simulink model "EKF_sim"  (R2020a)
settings: Solver=VariableStepAuto  StartTime=0.0  StopTime=257  RelTol=1e-3
values from neighbouring files (symbols this model uses):
  acc_variance = 4.8e-2    (= 0.048)    [init.m]
  bias_acc_variance = 4e-14    [init.m]
  bias_gyro_variance = 4e-14    [init.m]
  Delta2 = [260.168 -23.8158 1.64305]    [init.m]
  DT = EKF_DT    (= 0.01)    [init.m]
  EKF_DT = 0.01    [init.m]
  g = 9.81    [init.m]
  GPS_variance = 5    [init.m]
  gyro_variance = 4.8e-6    (= 4.8e-06)    [init.m]
  h0 = 38.8887000000000000    (= 38.8887)    [init.m]
  head_variance = 5e-2    (= 0.05)    [init.m]
  init_time = 4    [init.m]
  lambda_xa = 1e-4    (= 0.0001)    [init.m]
  lambda_xg = 1e-3    (= 0.001)    [init.m]
  lat0 = 36.7144590750000006    (= 36.714459075)    [init.m]
  lon0 = -4.4789588283333330    (= -4.47895882833)    [init.m]
  SHOE_buffer_N = 100    [init.m]
  SHOE_threshold = 2000    [init.m]
  t1_end = 100    [init.m]
  t1_start = 90    [init.m]
  t2_end = 193    [init.m]
  t2_start = 183    [init.m]
  t3_end = 213    [init.m]
  t3_start = 203    [init.m]
  t4_end = 244    [init.m]
  t4_start = 237    [init.m]
  type_of_GPS = 1    [init.m]
  vel_variance = 1e-2    (= 0.01)    [init.m]
  zero_vel_period = 0.1    [init.m]
(part 2 of 5)

== matlab function EKF_sim/EKF_nb/System Prediction/prediction_step ==
  data: x0 input; x_k output; P0 input; x_k_1 input size=16 1; P_k_1 input size=16 16; yg input; ya input; U input; P_k output size=16 16; DT parameter; g parameter; flag_init input; flag_init_ output
% --------------------         prediction           -------------------- %
%{
% This function computes the prediction step of the Kalman Filter. After 
% the initialization of the system, at each period the state vector is 
% updated, related to the prediction function and the measurement by the 
% inertial sensors (gyroscope and accelerometer). The covariance matrix P 
% is also updated.

% Input:
%     x0         : initial vector state
%     P0         : initial matrix P
%     x_k_1      : state vector before prediction step
%     P_k_1      : matrix P before prediction step
%     yg         : gyroscope measurement
%     ya         : accelerometer measurement
%     U          : covariance Matrix of input sensor
%     DT         : period of EKF system
%     g          : gravity acceleration
%     flag_init  : flag for initialization task

% Output:
%     x_k        : state vector after prediction step
%     P_k        : matrix P after prediction step
%     flag_init_ : flag for initialization task

% State vector x = [q w r v a]' [16x1]:
% q  = [q1 q2 q3 q4]     unit quaternion representing the attitude (1 2 3 4)
% w  = [wx wy wz]        angular velocity (5 6 7)
% r  = [rx ry rz]        position (NED)(8 9 10)
% v  = [vx vy vz]        linear velocity (NED) (11 12 13)
% a  = [ax ay az]        linear acceleration (NED) (14 15 16)
 
% Prediction model functions:
% fq = q * q(w*DT)
% fw = yg;
% fr = r + v*DT + a*DT*DT/2;
% fv = v + a*DT;
% fa = Rnb*ya + [0;0;g];

% P_k = Fx*P_k_1*Fx' + Fu*U*Fu'
 
% U = [gyro_variance(3x3),            0          
%        0                     acc_variance(3x3)]

% See 'calcolo_matrice_F_nb.m' for the exact calculation of matrices Fx and Fu
% These matrices are calculated offline, so note that if same parameters of 
% the system change, these matrices need to be changed.
%}
%%
function [x_k,  P_k, flag_init_] = prediction(x0, P0, x_k_1, P_k_1, ...
                                          yg, ya,...
                                          U, DT, g, flag_init)
    x_k = zeros(16,1);
    P_k = zeros(16,16);
    flag_init_ = flag_init;
    if flag_init ~= 0           %initialization check
        if flag_init == 1
            x_k_1 = x0;
            P_k_1 = P0;
            flag_init_ = 2;     %set flag=2 so the initialization is done
        end                     %one time only
        
        % Prediction Step
        [q_k_1,~,r_k_1,v_k_1,~] = extract_var(x_k_1);
        
        w_k  = yg;                                      %Velocity Rotation update with no bias compensation
        w_DT = (w_k*DT);                                %Angular displacement in DT time interval
        q_w  = new_q(w_DT(1),w_DT(2),w_DT(3));                        
        q    = q_product(q_k_1,q_w);                    %Rotations composition
        norm = (q(1)^2 + q(2)^2 + q(3)^2 + q(4)^2)^0.5;
        q_k  = q/norm;                                  %Normalize new quaternion
        Rnb  = fromq2rot(q_k(1),q_k(2),q_k(3),q_k(4));
       
        a_k  = Rnb*ya + [0;0;g];                        %Acceleration Update with no bias compensation
        v_k  = v_k_1 + a_k*DT;                          %Velocity update
        r_k  = r_k_1 + v_k*DT + a_k*DT*DT/2;            %Position update (origin of body frame)
        
        x_k = compact_var(q_k, w_k, r_k, v_k, a_k);          
        
        Fu = calcolo_Fu(q_k(1),q_k(2),q_k(3),q_k(4));
        Fx = calcolo_Fx(q_k(1),q_k(2),q_k(3),q_k(4),w_k(1),w_k(2),w_k(3),ya(1),ya(2),ya(3));
        P_k = Fx*P_k_1*Fx' + Fu*U*Fu';                  %Matrix P Update           
    end
end

%% Auxiliary Functions
% This function extracts single variables from the state vector
function [q, w, r, v, a] = extract_var(x)
    q  = x(1:4);
    w  = x(5:7);
    r  = x(8:10);
    v  = x(11:13);
    a  = x(14:16);
end

% This function compacts single variables into the state vector
function x = compact_var(q, w, r, v, a)
    x = zeros(16,1);
    x(1:4)   = q;
    x(5:7)   = w;
    x(8:10) =  r;
    x(11:13) = v;
    x(14:16) = a;
end

% This function computes the body-to-nav rotation matrix from quaternion
function rot = fromq2rot(q1,q2,q3,q4)
    rot = [q1^2+q2^2-q3^2-q4^2, 2*(q2*q3-q1*q4), 2*(q1*q3+q2*q4); ...
           2*(q2*q3+q1*q4), q1^2-q2^2+q3^2-q4^2, 2*(q3*q4-q1*q2); ...
           2*(q2*q4-q1*q3), 2*(q1*q2+q3*q4), q1^2-q2^2-q3^2+q4^2];
end

% This function create a quaternion from Euler's angle [Yaw,Pitch,Roll]
function q = new_q(yaw,pitch,roll)
    q = zeros(1,4);
    q(1) = cos(roll/2) * cos(pitch/2) * cos(yaw/2) + sin(roll/2) * sin(pitch/2) * sin(yaw/2);
    q(2) = sin(roll/2) * cos(pitch/2) * cos(yaw/2) - cos(roll/2) * sin(pitch/2) * sin(yaw/2);
    q(3) = cos(roll/2) * sin(pitch/2) * cos(yaw/2) + sin(roll/2) * cos(pitch/2) * sin(yaw/2);
    q(4) = cos(roll/2) * cos(pitch/2) * sin(yaw/2) - sin(roll/2) * sin(pitch/2) * cos(yaw/2);
    
end

% This function computes the product between two quaternion
function q = q_product(a,b)
    q = zeros(1,4);
    q(1) = b(1)*a(1) - b(2)*a(2) - b(3)*a(3) - b(4)*a(4);
    q(2) = b(1)*a(2) + b(2)*a(1) - b(3)*a(4) + b(4)*a(3);
    q(3) = b(1)*a(3) + b(2)*a(4) + b(3)*a(1) - b(4)*a(2);
    q(4) = b(1)*a(4) - b(2)*a(3) + b(3)*a(2) + b(4)*a(1);
end
%%
% These functions calculate the Fx and Fu matrices. 
% See 'calcolo_matrice_F_nb.m' for the symbolic calculation used
function Fx = calcolo_Fx(q1,q2,q3,q4,w_yaw,w_pitch,w_roll,ya1,ya2,ya3)
Fx =[(cos(w_pitch/200)*cos(w_roll/200)*cos(w_yaw/200) + sin(w_pitch/200)*sin(w_roll/200)*sin(w_yaw/200))/(q1^2 + q2^2 + q3^2 + q4^2)^(1/2) + (q1*(q2*(cos(w_pitch/200)*cos(w_yaw/200)*sin(w_roll/200) - cos(w_roll/200)*sin(w_pitch/200)*sin(w_yaw/200)) - q1*(cos(w_pitch/200)*cos(w_roll/200)*cos(w_yaw/200) + sin(w_pitch/200)*sin(w_roll/200)*sin(w_yaw/200)) + q3*(cos(w_roll/200)*cos(w_yaw/200)*sin(w_pitch/200) + cos(w_pitch/200)*sin(w_roll/200)*sin(w_yaw/200)) + q4*(cos(w_pitch/200)*cos(w_roll/200)*sin(w_yaw/200) - cos(w_yaw/200)*sin(w_pitch/200)*sin(w_roll/200))))/(q1^2 + q2^2 + q3^2 + q4^2)^(3/2),   (q2*(q2*(cos(w_pitch/200)*cos(w_yaw/200)*sin(w_roll/200) - cos(w_roll/200)*sin(w_pitch/200)*sin(w_yaw/200)) - q1*(cos(w_pitch/200)*cos(w_roll/200)*cos(w_yaw/200) + sin(w_pitch/200)*sin(w_roll/200)*sin(w_yaw/200)) + q3*(cos(w_roll/200)*cos(w_yaw/200)*sin(w_pitch/200) + cos(w_pitch/200)*sin(w_roll/200)*sin(w_yaw/200)) + q4*(cos(w_pitch/200)*cos(w_roll/200)*sin(w_yaw/200) - cos(w_yaw/200)*sin(w_pitch/200)*sin(w_roll/200))))/(q1^2 + q2^2 + q3^2 + q4^2)^(3/2) - (cos(w_pitch/200)*cos(w_yaw/200)*sin(w_roll/200) - cos(w_roll/200)*sin(w_pitch/200)*sin(w_yaw/200))/(q1^2 + q2^2 + q3^2 + q4^2)^(1/2),   (q3*(q2*(cos(w_pitch/200)*cos(w_yaw/200)*sin(w_roll/200) - cos(w_roll/200)*sin(w_pitch/200)*sin(w_yaw/200)) - q1*(cos(w_pitch/200)*cos(w_roll/200)*cos(w_yaw/200) + sin(w_pitch/200)*sin(w_roll/200)*sin(w_yaw/200)) + q3*(cos(w_roll/200)*cos(w_yaw/200)*sin(w_pitch/200) + cos(w_pitch/200)*sin(w_roll/200)*sin(w_yaw/200)) + q4*(cos(w_pitch/200)*cos(w_roll/200)*sin(w_yaw/200) - cos(w_yaw/200)*sin(w_pitch/200)*sin(w_roll/200))))/(q1^2 + q2^2 + q3^2 + q4^2)^(3/2) - (cos(w_roll/200)*cos(w_yaw/200)*sin(w_pitch/200) + cos(w_pitch/200)*sin(w_roll/200)*sin(w_yaw/200))/(q1^2 + q2^2 + q3^2 + q4^2)^(1/2),   (q4*(q2*(cos(w_pitch/200)*cos(w_yaw/200)*sin(w_roll/200) - cos(w_roll/200)*sin(w_pitch/200)*sin(w_yaw/200)) - q1*(cos(w_pitch/200)*cos(w_roll/200)*cos(w_yaw/200) + sin(w_pitch/200)*sin(w_roll/200)*sin(w_yaw/200)) + q3*(cos(w_roll/200)*cos(w_yaw/200)*sin(w_pitch/200) + cos(w_pitch/200)*sin(w_roll/200)*sin(w_yaw/200)) + q4*(cos(w_pitch/200)*cos(w_roll/200)*sin(w_yaw/200) - cos(w_yaw/200)*sin(w_pitch/200)*sin(w_roll/200))))/(q1^2 + q2^2 + q3^2 + q4^2)^(3/2) - (cos(w_pitch/200)*cos(w_roll/200)*sin(w_yaw/200) - cos(w_yaw/200)*sin(w_pitch/200)*sin(w_roll/200))/(q1^2 + q2^2 + q3^2 + q4^2)^(1/2), -(q1*((cos(w_pitch/200)*cos(w_roll/200)*sin(w_yaw/200))/200 - (cos(w_yaw/200)*sin(w_pitch/200)*sin(w_roll/200))/200) - q2*((cos(w_roll/200)*cos(w_yaw/200)*sin(w_pitch/200))/200 + (cos(w_pitch/200)*sin(w_roll/200)*sin(w_yaw/200))/200) + q3*((cos(w_pitch/200)*cos(w_yaw/200)*sin(w_roll/200))/200 - (cos(w_roll/200)*sin(w_pitch/200)*sin(w_yaw/200))/200) + q4*((cos(w_pitch/200)*cos(w_roll/200)*cos(w_yaw/200))/200 + (sin(w_pitch/200)*sin(w_roll/200)*sin(w_yaw/200))/200))/(q1^2 + q2^2 + q3^2 + q4^2)^(1/2), -(q1*((cos(w_roll/200)*cos(w_yaw/200)*sin(w_pitch/200))/200 - (cos(w_pitch/200)*sin(w_roll/200)*sin(w_yaw/200))/200) - q2*((cos(w_pitch/200)*cos(w_roll/200)*sin(w_yaw/200))/200 + (cos(w_yaw/200)*sin(w_pitch/200)*sin(w_roll/200))/200) + q3*((cos(w_pitch/200)*cos(w_roll/200)*cos(w_yaw/200))/200 - (sin(w_pitch/200)*sin(w_roll/200)*sin(w_yaw/200))/200) - q4*((cos(w_pitch/200)*cos(w_yaw/200)*sin(w_roll/200))/200 + (cos(w_roll/200)*sin(w_pitch/200)*sin(w_yaw/200))/200))/(q1^2 + q2^2 + q3^2 + q4^2)^(1/2), -(q1*((cos(w_pitch/200)*cos(w_yaw/200)*sin(w_roll/200))/200 - (cos(w_roll/200)*sin(w_pitch/200)*sin(w_yaw/200))/200) + q2*((cos(w_pitch/200)*cos(w_roll/200)*cos(w_yaw/200))/200 + (sin(w_pitch/200)*sin(w_roll/200)*sin(w_yaw/200))/200) + q3*((cos(w_pitch/200)*cos(w_roll/200)*sin(w_yaw/200))/200 - (cos(w_yaw/200)*sin(w_pitch/200)*sin(w_roll/200))/200) - q4*((cos(w_roll/200)*cos(w_yaw/200)*sin(w_pitch/200))/200 + (cos(w_pitch/200)*sin(w_roll/200)*sin(w_yaw/200))/200))/(q1^2 + q2^2 + q3^2 + q4^2)^(1/2), 0, 0, 0,     0,     0,     0,       0,       0,       0;
     (cos(w_pitch/200)*cos(w_yaw/200)*sin(w_roll/200) - cos(w_roll/200)*sin(w_pitch/200)*sin(w_yaw/200))/(q1^2 + q2^2 + q3^2 + q4^2)^(1/2) - (q1*(q1*(cos(w_pitch/200)*cos(w_yaw/200)*sin(w_roll/200) - cos(w_roll/200)*sin(w_pitch/200)*sin(w_yaw/200)) + q2*(cos(w_pitch/200)*cos(w_roll/200)*cos(w_yaw/200) + sin(w_pitch/200)*sin(w_roll/200)*sin(w_yaw/200)) + q3*(cos(w_pitch/200)*cos(w_roll/200)*sin(w_yaw/200) - cos(w_yaw/200)*sin(w_pitch/200)*sin(w_roll/200)) - q4*(cos(w_roll/200)*cos(w_yaw/200)*sin(w_pitch/200) + cos(w_pitch/200)*sin(w_roll/200)*sin(w_yaw/200))))/(q1^2 + q2^2 + q3^2 + q4^2)^(3/2),   (cos(w_pitch/200)*cos(w_roll/200)*cos(w_yaw/200) + sin(w_pitch/200)*sin(w_roll/200)*sin(w_yaw/200))/(q1^2 + q2^2 + q3^2 + q4^2)^(1/2) - (q2*(q1*(cos(w_pitch/200)*cos(w_yaw/200)*sin(w_roll/200) - cos(w_roll/200)*sin(w_pitch/200)*sin(w_yaw/200)) + q2*(cos(w_pitch/200)*cos(w_roll/200)*cos(w_yaw/200) + sin(w_pitch/200)*sin(w_roll/200)*sin(w_yaw/200)) + q3*(cos(w_pitch/200)*cos(w_roll/200)*sin(w_yaw/200) - cos(w_yaw/200)*sin(w_pitch/200)*sin(w_roll/200)) - q4*(cos(w_roll/200)*cos(w_yaw/200)*sin(w_pitch/200) + cos(w_pitch/200)*sin(w_roll/200)*sin(w_yaw/200))))/(q1^2 + q2^2 + q3^2 + q4^2)^(3/2),   (cos(w_pitch/200)*cos(w_roll/200)*sin(w_yaw/200) - cos(w_yaw/200)*sin(w_pitch/200)*sin(w_roll/200))/(q1^2 + q2^2 + q3^2 + q4^2)^(1/2) - (q3*(q1*(cos(w_pitch/200)*cos(w_yaw/200)*sin(w_roll/200) - cos(w_roll/200)*sin(w_pitch/200)*sin(w_yaw/200)) + q2*(cos(w_pitch/200)*cos(w_roll/200)*cos(w_yaw/200) + sin(w_pitch/200)*sin(w_roll/200)*sin(w_yaw/200)) + q3*(cos(w_pitch/200)*cos(w_roll/200)*sin(w_yaw/200) - cos(w_yaw/200)*sin(w_pitch/200)*sin(w_roll/200)) - q4*(cos(w_roll/200)*cos(w_yaw/200)*sin(w_pitch/200) + cos(w_pitch/200)*sin(w_roll/200)*sin(w_yaw/200))))/(q1^2 + q2^2 + q3^2 + q4^2)^(3/2), - (cos(w_roll/200)*cos(w_yaw/200)*sin(w_pitch/200) + cos(w_pitch/200)*sin(w_roll/200)*sin(w_yaw/200))/(q1^2 + q2^2 + q3^2 + q4^2)^(1/2) - (q4*(q1*(cos(w_pitch/200)*cos(w_yaw/200)*sin(w_roll/200) - cos(w_roll/200)*sin(w_pitch/200)*sin(w_yaw/200)) + q2*(cos(w_pitch/200)*cos(w_roll/200)*cos(w_yaw/200) + sin(w_pitch/200)*sin(w_roll/200)*sin(w_yaw/200)) + q3*(cos(w_pitch/200)*cos(w_roll/200)*sin(w_yaw/200) - cos(w_yaw/200)*sin(w_pitch/200)*sin(w_roll/200)) - q4*(cos(w_roll/200)*cos(w_yaw/200)*sin(w_pitch/200) + cos(w_pitch/200)*sin(w_roll/200)*sin(w_yaw/200))))/(q1^2 + q2^2 + q3^2 + q4^2)^(3/2), -(q1*((cos(w_roll/200)*cos(w_yaw/200)*sin(w_pitch/200))/200 + (cos(w_pitch/200)*sin(w_roll/200)*sin(w_yaw/200))/200) + q2*((cos(w_pitch/200)*cos(w_roll/200)*sin(w_yaw/200))/200 - (cos(w_yaw/200)*sin(w_pitch/200)*sin(w_roll/200))/200) - q3*((cos(w_pitch/200)*cos(w_roll/200)*cos(w_yaw/200))/200 + (sin(w_pitch/200)*sin(w_roll/200)*sin(w_yaw/200))/200) + q4*((cos(w_pitch/200)*cos(w_yaw/200)*sin(w_roll/200))/200 - (cos(w_roll/200)*sin(w_pitch/200)*sin(w_yaw/200))/200))/(q1^2 + q2^2 + q3^2 + q4^2)^(1/2), -(q1*((cos(w_pitch/200)*cos(w_roll/200)*sin(w_yaw/200))/200 + (cos(w_yaw/200)*sin(w_pitch/200)*sin(w_roll/200))/200) + q2*((cos(w_roll/200)*cos(w_yaw/200)*sin(w_pitch/200))/200 - (cos(w_pitch/200)*sin(w_roll/200)*sin(w_yaw/200))/200) + q3*((cos(w_pitch/200)*cos(w_yaw/200)*sin(w_roll/200))/200 + (cos(w_roll/200)*sin(w_pitch/200)*sin(w_yaw/200))/200) + q4*((cos(w_pitch/200)*cos(w_roll/200)*cos(w_yaw/200))/200 - (sin(w_pitch/200)*sin(w_roll/200)*sin(w_yaw/200))/200))/(q1^2 + q2^2 + q3^2 + q4^2)^(1/2), -(q2*((cos(w_pitch/200)*cos(w_yaw/200)*sin(w_roll/200))/200 - (cos(w_roll/200)*sin(w_pitch/200)*sin(w_yaw/200))/200) - q1*((cos(w_pitch/200)*cos(w_roll/200)*cos(w_yaw/200))/200 + (sin(w_pitch/200)*sin(w_roll/200)*sin(w_yaw/200))/200) + q3*((cos(w_roll/200)*cos(w_yaw/200)*sin(w_pitch/200))/200 + (cos(w_pitch/200)*sin(w_roll/200)*sin(w_yaw/200))/200) + q4*((cos(w_pitch/200)*cos(w_roll/200)*sin(w_yaw/200))/200 - (cos(w_yaw/200)*sin(w_pitch/200)*sin(w_roll/200))/200))/(q1^2 + q2^2 + q3^2 + q4^2)^(1/2), 0, 0, 0,     0,     0,     0,       0,       0,       0;
     (cos(w_roll/200)*cos(w_yaw/200)*sin(w_pitch/200) + cos(w_pitch/200)*sin(w_roll/200)*sin(w_yaw/200))/(q1^2 + q2^2 + q3^2 + q4^2)^(1/2) - (q1*(q1*(cos(w_roll/200)*cos(w_yaw/200)*sin(w_pitch/200) + cos(w_pitch/200)*sin(w_roll/200)*sin(w_yaw/200)) - q2*(cos(w_pitch/200)*cos(w_roll/200)*sin(w_yaw/200) - cos(w_yaw/200)*sin(w_pitch/200)*sin(w_roll/200)) + q3*(cos(w_pitch/200)*cos(w_roll/200)*cos(w_yaw/200) + sin(w_pitch/200)*sin(w_roll/200)*sin(w_yaw/200)) + q4*(cos(w_pitch/200)*cos(w_yaw/200)*sin(w_roll/200) - cos(w_roll/200)*sin(w_pitch/200)*sin(w_yaw/200))))/(q1^2 + q2^2 + q3^2 + q4^2)^(3/2), - (cos(w_pitch/200)*cos(w_roll/200)*sin(w_yaw/200) - cos(w_yaw/200)*sin(w_pitch/200)*sin(w_roll/200))/(q1^2 + q2^2 + q3^2 + q4^2)^(1/2) - (q2*(q1*(cos(w_roll/200)*cos(w_yaw/200)*sin(w_pitch/200) + cos(w_pitch/200)*sin(w_roll/200)*sin(w_yaw/200)) - q2*(cos(w_pitch/200)*cos(w_roll/200)*sin(w_yaw/200) - cos(w_yaw/200)*sin(w_pitch/200)*sin(w_roll/200)) + q3*(cos(w_pitch/200)*cos(w_roll/200)*cos(w_yaw/200) + sin(w_pitch/200)*sin(w_roll/200)*sin(w_yaw/200)) + q4*(cos(w_pitch/200)*cos(w_yaw/200)*sin(w_roll/200) - cos(w_roll/200)*sin(w_pitch/200)*sin(w_yaw/200))))/(q1^2 + q2^2 + q3^2 + q4^2)^(3/2),   (cos(w_pitch/200)*cos(w_roll/200)*cos(w_yaw/200) + sin(w_pitch/200)*sin(w_roll/200)*sin(w_yaw/200))/(q1^2 + q2^2 + q3^2 + q4^2)^(1/2) - (q3*(q1*(cos(w_roll/200)*cos(w_yaw/200)*sin(w_pitch/200) + cos(w_pitch/200)*sin(w_roll/200)*sin(w_yaw/200)) - q2*(cos(w_pitch/200)*cos(w_roll/200)*sin(w_yaw/200) - cos(w_yaw/200)*sin(w_pitch/200)*sin(w_roll/200)) + q3*(cos(w_pitch/200)*cos(w_roll/200)*cos(w_yaw/200) + sin(w_pitch/200)*sin(w_roll/200)*sin(w_yaw/200)) + q4*(cos(w_pitch/200)*cos(w_yaw/200)*sin(w_roll/200) - cos(w_roll/200)*sin(w_pitch/200)*sin(w_yaw/200))))/(q1^2 + q2^2 + q3^2 + q4^2)^(3/2),   (cos(w_pitch/200)*cos(w_yaw/200)*sin(w_roll/200) - cos(w_roll/200)*sin(w_pitch/200)*sin(w_yaw/200))/(q1^2 + q2^2 + q3^2 + q4^2)^(1/2) - (q4*(q1*(cos(w_roll/200)*cos(w_yaw/200)*sin(w_pitch/200) + cos(w_pitch/200)*sin(w_roll/200)*sin(w_yaw/200)) - q2*(cos(w_pitch/200)*cos(w_roll/200)*sin(w_yaw/200) - cos(w_yaw/200)*sin(w_pitch/200)*sin(w_roll/200)) + q3*(cos(w_pitch/200)*cos(w_roll/200)*cos(w_yaw/200) + sin(w_pitch/200)*sin(w_roll/200)*sin(w_yaw/200)) + q4*(cos(w_pitch/200)*cos(w_yaw/200)*sin(w_roll/200) - cos(w_roll/200)*sin(w_pitch/200)*sin(w_yaw/200))))/(q1^2 + q2^2 + q3^2 + q4^2)^(3/2), -(q2*((cos(w_pitch/200)*cos(w_roll/200)*cos(w_yaw/200))/200 + (sin(w_pitch/200)*sin(w_roll/200)*sin(w_yaw/200))/200) - q1*((cos(w_pitch/200)*cos(w_yaw/200)*sin(w_roll/200))/200 - (cos(w_roll/200)*sin(w_pitch/200)*sin(w_yaw/200))/200) + q3*((cos(w_pitch/200)*cos(w_roll/200)*sin(w_yaw/200))/200 - (cos(w_yaw/200)*sin(w_pitch/200)*sin(w_roll/200))/200) + q4*((cos(w_roll/200)*cos(w_yaw/200)*sin(w_pitch/200))/200 + (cos(w_pitch/200)*sin(w_roll/200)*sin(w_yaw/200))/200))/(q1^2 + q2^2 + q3^2 + q4^2)^(1/2),  (q1*((cos(w_pitch/200)*cos(w_roll/200)*cos(w_yaw/200))/200 - (sin(w_pitch/200)*sin(w_roll/200)*sin(w_yaw/200))/200) + q2*((cos(w_pitch/200)*cos(w_yaw/200)*sin(w_roll/200))/200 + (cos(w_roll/200)*sin(w_pitch/200)*sin(w_yaw/200))/200) - q3*((cos(w_roll/200)*cos(w_yaw/200)*sin(w_pitch/200))/200 - (cos(w_pitch/200)*sin(w_roll/200)*sin(w_yaw/200))/200) - q4*((cos(w_pitch/200)*cos(w_roll/200)*sin(w_yaw/200))/200 + (cos(w_yaw/200)*sin(w_pitch/200)*sin(w_roll/200))/200))/(q1^2 + q2^2 + q3^2 + q4^2)^(1/2),  (q1*((cos(w_pitch/200)*cos(w_roll/200)*sin(w_yaw/200))/200 - (cos(w_yaw/200)*sin(w_pitch/200)*sin(w_roll/200))/200) + q2*((cos(w_roll/200)*cos(w_yaw/200)*sin(w_pitch/200))/200 + (cos(w_pitch/200)*sin(w_roll/200)*sin(w_yaw/200))/200) - q3*((cos(w_pitch/200)*cos(w_yaw/200)*sin(w_roll/200))/200 - (cos(w_roll/200)*sin(w_pitch/200)*sin(w_yaw/200))/200) + q4*((cos(w_pitch/200)*cos(w_roll/200)*cos(w_yaw/200))/200 + (sin(w_pitch/200)*sin(w_roll/200)*sin(w_yaw/200))/200))/(q1^2 + q2^2 + q3^2 + q4^2)^(1/2), 0, 0, 0,     0,     0,     0,       0,       0,       0;
     (cos(w_pitch/200)*cos(w_roll/200)*sin(w_yaw/200) - cos(w_yaw/200)*sin(w_pitch/200)*sin(w_roll/200))/(q1^2 + q2^2 + q3^2 + q4^2)^(1/2) - (q1*(q1*(cos(w_pitch/200)*cos(w_roll/200)*sin(w_yaw/200) - cos(w_yaw/200)*sin(w_pitch/200)*sin(w_roll/200)) + q2*(cos(w_roll/200)*cos(w_yaw/200)*sin(w_pitch/200) + cos(w_pitch/200)*sin(w_roll/200)*sin(w_yaw/200)) - q3*(cos(w_pitch/200)*cos(w_yaw/200)*sin(w_roll/200) - cos(w_roll/200)*sin(w_pitch/200)*sin(w_yaw/200)) + q4*(cos(w_pitch/200)*cos(w_roll/200)*cos(w_yaw/200) + sin(w_pitch/200)*sin(w_roll/200)*sin(w_yaw/200))))/(q1^2 + q2^2 + q3^2 + q4^2)^(3/2),   (cos(w_roll/200)*cos(w_yaw/200)*sin(w_pitch/200) + cos(w_pitch/200)*sin(w_roll/200)*sin(w_yaw/200))/(q1^2 + q2^2 + q3^2 + q4^2)^(1/2) - (q2*(q1*(cos(w_pitch/200)*cos(w_roll/200)*sin(w_yaw/200) - cos(w_yaw/200)*sin(w_pitch/200)*sin(w_roll/200)) + q2*(cos(w_roll/200)*cos(w_yaw/200)*sin(w_pitch/200) + cos(w_pitch/200)*sin(w_roll/200)*sin(w_yaw/200)) - q3*(cos(w_pitch/200)*cos(w_yaw/200)*sin(w_roll/200) - cos(w_roll/200)*sin(w_pitch/200)*sin(w_yaw/200)) + q4*(cos(w_pitch/200)*cos(w_roll/200)*cos(w_yaw/200) + sin(w_pitch/200)*sin(w_roll/200)*sin(w_yaw/200))))/(q1^2 + q2^2 + q3^2 + q4^2)^(3/2), - (cos(w_pitch/200)*cos(w_yaw/200)*sin(w_roll/200) - cos(w_roll/200)*sin(w_pitch/200)*sin(w_yaw/200))/(q1^2 + q2^2 + q3^2 + q4^2)^(1/2) - (q3*(q1*(cos(w_pitch/200)*cos(w_roll/200)*sin(w_yaw/200) - cos(w_yaw/200)*sin(w_pitch/200)*sin(w_roll/200)) + q2*(cos(w_roll/200)*cos(w_yaw/200)*sin(w_pitch/200) + cos(w_pitch/200)*sin(w_roll/200)*sin(w_yaw/200)) - q3*(cos(w_pitch/200)*cos(w_yaw/200)*sin(w_roll/200) - cos(w_roll/200)*sin(w_pitch/200)*sin(w_yaw/200)) + q4*(cos(w_pitch/200)*cos(w_roll/200)*cos(w_yaw/200) + sin(w_pitch/200)*sin(w_roll/200)*sin(w_yaw/200))))/(q1^2 + q2^2 + q3^2 + q4^2)^(3/2),   (cos(w_pitch/200)*cos(w_roll/200)*cos(w_yaw/200) + sin(w_pitch/200)*sin(w_roll/200)*sin(w_yaw/200))/(q1^2 + q2^2 + q3^2 + q4^2)^(1/2) - (q4*(q1*(cos(w_pitch/200)*cos(w_roll/200)*sin(w_yaw/200) - cos(w_yaw/200)*sin(w_pitch/200)*sin(w_roll/200)) + q2*(cos(w_roll/200)*cos(w_yaw/200)*sin(w_pitch/200) + cos(w_pitch/200)*sin(w_roll/200)*sin(w_yaw/200)) - q3*(cos(w_pitch/200)*cos(w_yaw/200)*sin(w_roll/200) - cos(w_roll/200)*sin(w_pitch/200)*sin(w_yaw/200)) + q4*(cos(w_pitch/200)*cos(w_roll/200)*cos(w_yaw/200) + sin(w_pitch/200)*sin(w_roll/200)*sin(w_yaw/200))))/(q1^2 + q2^2 + q3^2 + q4^2)^(3/2),  (q1*((cos(w_pitch/200)*cos(w_roll/200)*cos(w_yaw/200))/200 + (sin(w_pitch/200)*sin(w_roll/200)*sin(w_yaw/200))/200) + q2*((cos(w_pitch/200)*cos(w_yaw/200)*sin(w_roll/200))/200 - (cos(w_roll/200)*sin(w_pitch/200)*sin(w_yaw/200))/200) + q3*((cos(w_roll/200)*cos(w_yaw/200)*sin(w_pitch/200))/200 + (cos(w_pitch/200)*sin(w_roll/200)*sin(w_yaw/200))/200) - q4*((cos(w_pitch/200)*cos(w_roll/200)*sin(w_yaw/200))/200 - (cos(w_yaw/200)*sin(w_pitch/200)*sin(w_roll/200))/200))/(q1^2 + q2^2 + q3^2 + q4^2)^(1/2), -(q1*((cos(w_pitch/200)*cos(w_yaw/200)*sin(w_roll/200))/200 + (cos(w_roll/200)*sin(w_pitch/200)*sin(w_yaw/200))/200) - q2*((cos(w_pitch/200)*cos(w_roll/200)*cos(w_yaw/200))/200 - (sin(w_pitch/200)*sin(w_roll/200)*sin(w_yaw/200))/200) - q3*((cos(w_pitch/200)*cos(w_roll/200)*sin(w_yaw/200))/200 + (cos(w_yaw/200)*sin(w_pitch/200)*sin(w_roll/200))/200) + q4*((cos(w_roll/200)*cos(w_yaw/200)*sin(w_pitch/200))/200 - (cos(w_pitch/200)*sin(w_roll/200)*sin(w_yaw/200))/200))/(q1^2 + q2^2 + q3^2 + q4^2)^(1/2), -(q1*((cos(w_roll/200)*cos(w_yaw/200)*sin(w_pitch/200))/200 + (cos(w_pitch/200)*sin(w_roll/200)*sin(w_yaw/200))/200) - q2*((cos(w_pitch/200)*cos(w_roll/200)*sin(w_yaw/200))/200 - (cos(w_yaw/200)*sin(w_pitch/200)*sin(w_roll/200))/200) + q3*((cos(w_pitch/200)*cos(w_roll/200)*cos(w_yaw/200))/200 + (sin(w_pitch/200)*sin(w_roll/200)*sin(w_yaw/200))/200) + q4*((cos(w_pitch/200)*cos(w_yaw/200)*sin(w_roll/200))/200 - (cos(w_roll/200)*sin(w_pitch/200)*sin(w_yaw/200))/200))/(q1^2 + q2^2 + q3^2 + q4^2)^(1/2), 0, 0, 0,     0,     0,     0,       0,       0,       0;
                                                                                                                                                                                                                                                                                                                                                                                                                                                                                                                                                                                                                      0,                                                                                                                                                                                                                                                                                                                                                                                                                                                                                                                                                                                                                    0,                                                                                                                                                                                                                                                                                                                                                                                                                                                                                                                                                                                                                    0,                                                                                                                                                                                                                                                                                                                                                                                                                                                                                                                                                                                                                    0,                                                                                                                                                                                                                                                                                                                                                                                                                                                                                                                      0,                                                                                                                                                                                                                                                                                                                                                                                                                                                                                                                      0,                                                                                                                                                                                                                                                                                                                                                                                                                                                                                                                      0, 0, 0, 0,     0,     0,     0,       0,       0,       0;
                                                                                                                                                                                                                                                                                                                                                                                                                                                                                                                                                                                                                      0,                                                                                                                                                                                                                                                                                                                                                                                                                                                                                                                                                                                                                    0,                                                                                                                                                                                                                                                                                                                                                                                                                                                                                                                                                                                                                    0,                                                                                                                                                                                                                                                                                                                                                                                                                                                                                                                                                                                                                    0,                                                                                                                                                                                                                                                                                                                                                                                                                                                                                                                      0,                                                                                                                                                                                                                                                                                                                                                                                                                                                                                                                      0,                                                                                                                                                                                                                                                                                                                                                                                                                                                                                                                      0, 0, 0, 0,     0,     0,     0,       0,       0,       0;
                                                                                                                                                                                                                                                                                                                                                                                                                                                                                                                                                                                                                      0,                                                                                                                                                                                                                                                                                                                                                                                                                                                                                                                                                                                                                    0,                                                                                                                                                                                                                                                                                                                                                                                                                                                                                                                                                                                                                    0,                                                                                                                                                                                                                                                                                                                                                                                                                                                                                                                                                                                                                    0,                                                                                                                                                                                                                                                                                                                                                                                                                                                                                                                      0,                                                                                                                                                                                                                                                                                                                                                                                                                                                                                                                      0,                                                                                                                                                                                                                                                                                                                                                                                                                                                                                                                      0, 0, 0, 0,     0,     0,     0,       0,       0,       0;
                                                                                                                                                                                                                                                                                                                                                                                                                                                                                                                                                                                                                      0,                                                                                                                                                                                                                                                                                                                                                                                                                                                                                                                                                                                                                    0,                                                                                                                                                                                                                                                                                                                                                                                                                                                                                                                                                                                                                    0,                                                                                                                                                                                                                                                                                                                                                                                                                                                                                                                                                                                                                    0,                                                                                                                                                                                                                                                                                                                                                                                                                                                                                                                      0,                                                                                                                                                                                                                                                                                                                                                                                                                                                                                                                      0,                                                                                                                                                                                                                                                                                                                                                                                                                                                                                                                      0, 1, 0, 0, 1/100,     0,     0, 1/20000,       0,       0;
                                                                                                                                                                                                                                                                                                                                                                                                                                                                                                                                                                                                                      0,                                                                                                                                                                                                                                                                                                                                                                                                                                                                                                                                                                                                                    0,                                                                                                                                                                                                                                                                                                                                                                                                                                                                                                                                                                                                                    0,                                                                                                                                                                                                                                                                                                                                                                                                                                                                                                                                                                                                                    0,                                                                                                                                                                                                                                                                                                                                                                                                                                                                                                                      0,                                                                                                                                                                                                                                                                                                                                                                                                                                                                                                                      0,                                                                                                                                                                                                                                                                                                                                                                                                                                                                                                                      0, 0, 1, 0,     0, 1/100,     0,       0, 1/20000,       0;
                                                                                                                                                                                                                                                                                                                                                                                                                                                                                                                                                                                                                      0,                                                                                                                                                                                                                                                                                                                                                                                                                                                                                                                                                                                                                    0,                                                                                                                                                                                                                                                                                                                                                                                                                                                                                                                                                                                                                    0,                                                                                                                                                                                                                                                                                                                                                                                                                                                                                                                                                                                                                    0,                                                                                                                                                                                                                                                                                                                                                                                                                                                                                                                      0,                                                                                                                                                                                                                                                                                                                                                                                                                                                                                                                      0,                                                                                                                                                                                                                                                                                                                                                                                                                                                                                                                      0, 0, 0, 1,     0,     0, 1/100,       0,       0, 1/20000;
                                                                                                                                                                                                                                                                                                                                                                                                                                                                                                                                                                                                                      0,                                                                                                                                                                                                                                                                                                                                                                                                                                                                                                                                                                                                                    0,                                                                                                                                                                                                                                                                                                                                                                                                                                                                                                                                                                                                                    0,                                                                                                                                                                                                                                                                                                                                                                                                                                                                                                                                                                                                                    0,                                                                                                                                                                                                                                                                                                                                                                                                                                                                                                                      0,                                                                                                                                                                                                                                                                                                                                                                                                                                                                                                                      0,                                                                                                                                                                                                                                                                                                                                                                                                                                                                                                                      0, 0, 0, 0,     1,     0,     0,   1/100,       0,       0;
                                                                                                                                                                                                                                                                                                                                                                                                                                                                                                                                                                                                                      0,                                                                                                                                                                                                                                                                                                                                                                                                                                                                                                                                                                                                                    0,                                                                                                                                                                                                                                                                                                                                                                                                                                                                                                                                                                                                                    0,                                                                                                                                                                                                                                                                                                                                                                                                                                                                                                                                                                                                                    0,                                                                                                                                                                                                                                                                                                                                                                                                                                                                                                                      0,                                                                                                                                                                                                                                                                                                                                                                                                                                                                                                                      0,                                                                                                                                                                                                                                                                                                                                                                                                                                                                                                                      0, 0, 0, 0,     0,     1,     0,       0,   1/100,       0;
                                                                                                                                                                                                                                                                                                                                                                                                                                                                                                                                                                                                                      0,                                                                                                                                                                                                                                                                                                                                                                                                                                                                                                                                                                                                                    0,                                                                                                                                                                                                                                                                                                                                                                                                                                                                                                                                                                                                                    0,                                                                                                                                                                                                                                                                                                                                                                                                                                                                                                                                                                                                                    0,                                                                                                                                                                                                                                                                                                                                                                                                                                                                                                                      0,                                                                                                                                                                                                                                                                                                                                                                                                                                                                                                                      0,                                                                                                                                                                                                                                                                                                                                                                                                                                                                                                                      0, 0, 0, 0,     0,     0,     1,       0,       0,   1/100;
                                                                                                                                                                                                                                                                                                                                                                                                                                                                                                                                                                                         2*q1*ya1 + 2*q3*ya3 - 2*q4*ya2,                                                                                                                                                                                                                                                                                                                                                                                                                                                                                                                                                                                       2*q2*ya1 + 2*q3*ya2 + 2*q4*ya3,                                                                                                                                                                                                                                                                                                                                                                                                                                                                                                                                                                                       2*q1*ya3 + 2*q2*ya2 - 2*q3*ya1,                                                                                                                                                                                                                                                                                                                                                                                                                                                                                                                                                                                       2*q2*ya3 - 2*q1*ya2 - 2*q4*ya1,                                                                                                                                                                                                                                                                                                                                                                                                                                                                                                                      0,                                                                                                                                                                                                                                                                                                                                                                                                                                                                                                                      0,                                                                                                                                                                                                                                                                                                                                                                                                                                                                                                                      0, 0, 0, 0,     0,     0,     0,       0,       0,       0;
                                                                                                                                                                                                                                                                                                                                                                                                                                                                                                                                                                                         2*q1*ya2 - 2*q2*ya3 + 2*q4*ya1,                                                                                                                                                                                                                                                                                                                                                                                                                                                                                                                                                                                       2*q3*ya1 - 2*q2*ya2 - 2*q1*ya3,                                                                                                                                                                                                                                                                                                                                                                                                                                                                                                                                                                                       2*q2*ya1 + 2*q3*ya2 + 2*q4*ya3,                                                                                                                                                                                                                                                                                                                                                                                                                                                                                                                                                                                       2*q1*ya1 + 2*q3*ya3 - 2*q4*ya2,                                                                                                                                                                                                                                                                                                                                                                                                                                                                                                                      0,                                                                                                                                                                                                                                                                                                                                                                                                                                                                                                                      0,                                                                                                                                                                                                                                                                                                                                                                                                                                                                                                                      0, 0, 0, 0,     0,     0,     0,       0,       0,       0;
                                                                                                                                                                                                                                                                                                                                                                                                                                                                                                                                                                                         2*q1*ya3 + 2*q2*ya2 - 2*q3*ya1,                                                                                                                                                                                                                                                                                                                                                                                                                                                                                                                                                                                       2*q1*ya2 - 2*q2*ya3 + 2*q4*ya1,                                                                                                                                                                                                                                                                                                                                                                                                                                                                                                                                                                                       2*q4*ya2 - 2*q3*ya3 - 2*q1*ya1,                                                                                                                                                                                                                                                                                                                                                                                                                                                                                                                                                                                       2*q2*ya1 + 2*q3*ya2 + 2*q4*ya3,                                                                                                                                                                                                                                                                                                                                                                                                                                                                                                                      0,                                                                                                                                                                                                                                                                                                                                                                                                                                                                                                                      0,                                                                                                                                                                                                                                                                                                                                                                                                                                                                                                                      0, 0, 0, 0,     0,     0,     0,       0,       0,       0];

end

function Fu = calcolo_Fu(q1,q2,q3,q4)
Fu =[0, 0, 0,                         0,                         0,                         0;
     0, 0, 0,                         0,                         0,                         0;
     0, 0, 0,                         0,                         0,                         0;
     0, 0, 0,                         0,                         0,                         0;
     1, 0, 0,                         0,                         0,                         0;
     0, 1, 0,                         0,                         0,                         0;
     0, 0, 1,                         0,                         0,                         0;
     0, 0, 0,                         0,                         0,                         0;
     0, 0, 0,                         0,                         0,                         0;
     0, 0, 0,                         0,                         0,                         0;
     0, 0, 0,                         0,                         0,                         0;
     0, 0, 0,                         0,                         0,                         0;
     0, 0, 0,                         0,                         0,                         0;
     0, 0, 0, q1^2 + q2^2 - q3^2 - q4^2,         2*q2*q3 - 2*q1*q4,         2*q1*q3 + 2*q2*q4;
     0, 0, 0,         2*q1*q4 + 2*q2*q3, q1^2 - q2^2 + q3^2 - q4^2,         2*q3*q4 - 2*q1*q2;
     0, 0, 0,         2*q2*q4 - 2*q1*q3,         2*q1*q2 + 2*q3*q4, q1^2 - q2^2 - q3^2 + q4^2];
end

%% %%%%%%%%%%%%%%%%%%%%%%%%%%%%%%%%%%%%%%%%%%%%%%%%%%%%%%%%%%%%%%%%%%%%%%%
     %%%%%%%%% Direct EKF for 6D Pose,  Marco Borraccino %%%%%%%%%%
     %%%%%%%%%   SGN Project, University of Pisa, 2021   %%%%%%%%%%
%%%%%%%%%%%%%%%%%%%%%%%%%%%%%%%%%%%%%%%%%%%%%%%%%%%%%%%%%%%%%%%%%%%%%%%%%%
